simulink model "COMPENSATED"  (R2022b)
settings: Solver=VariableStepAuto  StartTime=0.0  StopTime=0.001  RelTol=1e-3
libraries: spsSeriesRLCBranchLib x9, spsDiodeLib x4, spsIGBTDiodeLib x4, spsCurrentMeasurementLib x3, spsVoltageMeasurementLib x3, spsDCVoltageSourceLib x1, spsPWMGeneratorDCDCLib x1, spspowerguiLib x1
settings Model: Creator=Hafeni  LastModifiedBy=Hafeni

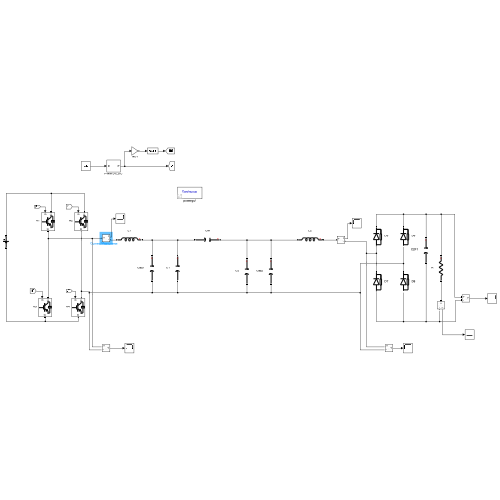
[thumbnail: Simulink's stored preview of the top-level diagram]
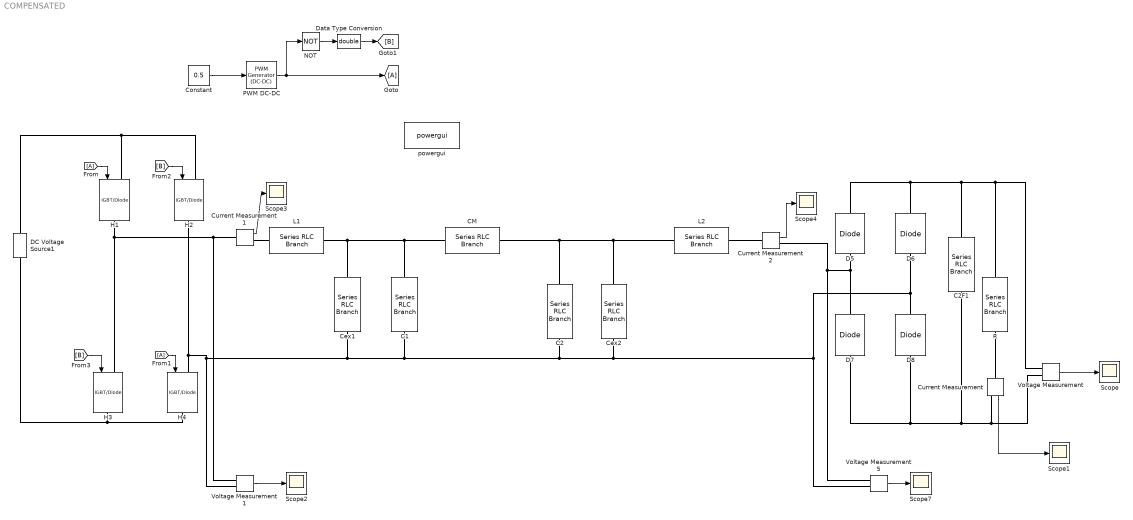
== system COMPENSATED ==
  C1 : spsSeriesRLCBranchLib/Series RLC Branch  LConnTagsString=__new0  RConnTagsString=__new0  BranchType=C  Resistance=1e-6  Inductance=1e-3  SetiL0=off  InitialCurrent=0  Capacitance=1.6460e-12  Setx0=off  InitialVoltage=0  Measurements=Branch voltage
  C2 : spsSeriesRLCBranchLib/Series RLC Branch  LConnTagsString=__new0  RConnTagsString=__new0  BranchType=C  Resistance=1e-6  Inductance=1e-3  SetiL0=off  InitialCurrent=0  Capacitance=1.6456e-12  Setx0=off  InitialVoltage=0  Measurements=Branch voltage
  C2F1 : spsSeriesRLCBranchLib/Series RLC Branch  LConnTagsString=__new0  RConnTagsString=__new0  BranchType=C  Resistance=1e-6  Inductance=1e-3  SetiL0=off  InitialCurrent=0  Capacitance=10e-6  Setx0=off  InitialVoltage=0  Measurements=Branch voltage
  CM : spsSeriesRLCBranchLib/Series RLC Branch  LConnTagsString=__new0  RConnTagsString=__new0  BranchType=C  Resistance=1e-6  Inductance=1e-3  SetiL0=off  InitialCurrent=0  Capacitance=1.0341e-10  Setx0=off  InitialVoltage=0  Measurements=Branch voltage
  Cex1 : spsSeriesRLCBranchLib/Series RLC Branch  LConnTagsString=__new0  RConnTagsString=__new0  BranchType=C  Resistance=1e-6  Inductance=1e-3  SetiL0=off  InitialCurrent=0  Capacitance=100e-12  Setx0=off  InitialVoltage=0  Measurements=Branch voltage
  Cex2 : spsSeriesRLCBranchLib/Series RLC Branch  LConnTagsString=__new0  RConnTagsString=__new0  BranchType=C  Resistance=1e-6  Inductance=1e-3  SetiL0=off  InitialCurrent=0  Capacitance=100e-12  Setx0=off  InitialVoltage=0  Measurements=Branch voltage
  Constant : Constant  Value=0.5
  Current Measurement : spsCurrentMeasurementLib/Current Measurement  PhasorSimulation=off  OutputType=Complex  PSBequivalent=0
  Current Measurement1 : spsCurrentMeasurementLib/Current Measurement  PhasorSimulation=off  OutputType=Complex  PSBequivalent=0
  Current Measurement2 : spsCurrentMeasurementLib/Current Measurement  PhasorSimulation=off  OutputType=Complex  PSBequivalent=0
  D{5..8} (4 alike) : spsDiodeLib/Diode  Ron=0.001  Lon=0  Vf=0.8  IC=0  UseSnubber=0  Rs=500  Cs=250e-9  Measurements=off
  DC Voltage Source1 : spsDCVoltageSourceLib/DC Voltage Source  Amplitude=12  Measurements=None
  Data Type Conversion : DataTypeConversion  OutDataTypeStr=double  SaturateOnIntegerOverflow=off  RndMeth=Floor
  From : From
  From1 : From
  Goto : Goto
  H{1..4} (4 alike) : spsIGBTDiodeLib/IGBT//Diode  Ron=1e-3  Rs=1e5  Cs=inf  Measurements=off
  L1 : spsSeriesRLCBranchLib/Series RLC Branch  LConnTagsString=__new0  RConnTagsString=__new0  BranchType=L  Resistance=1e-6  Inductance=1.38e-6  SetiL0=off  InitialCurrent=0  Capacitance=1.0341e-10  Setx0=off  InitialVoltage=0  Measurements=Branch voltage
  L2 : spsSeriesRLCBranchLib/Series RLC Branch  LConnTagsString=__new0  RConnTagsString=__new0  BranchType=L  Resistance=1e-6  Inductance=1.38e-6  SetiL0=off  InitialCurrent=0  Capacitance=1.0341e-10  Setx0=off  InitialVoltage=0  Measurements=Branch voltage
  "NOT " : Logic  Operator=NOT  IconShape=distinctive  AllPortsSameDT=off  OutDataTypeStr=boolean
  PWM DC-DC : spsPWMGeneratorDCDCLib/PWM Generator (DC-DC)  Fsw=13560000  Ts=0
  R : spsSeriesRLCBranchLib/Series RLC Branch  LConnTagsString=__new0  RConnTagsString=__new0  BranchType=R  Resistance=3.04  Inductance=1e-3  SetiL0=off  InitialCurrent=0  Capacitance=300e-6  Setx0=off  InitialVoltage=0  Measurements=Branch voltage
  Scope{,1..4,7} (6 alike) : Scope
  Voltage Measurement : spsVoltageMeasurementLib/Voltage Measurement  PhasorSimulation=off  OutputType=Complex  PSBequivalent=0
  Voltage Measurement1 : spsVoltageMeasurementLib/Voltage Measurement  PhasorSimulation=off  OutputType=Complex  PSBequivalent=0
  Voltage Measurement5 : spsVoltageMeasurementLib/Voltage Measurement  PhasorSimulation=off  OutputType=Complex  PSBequivalent=0
  powergui : spspowerguiLib/powergui  Priority=1  SimulationMode=Continuous  SampleTime=50e-6  frequency=60  Iterations=50  frequencyindice=0  Pbase=100e6  ErrMax=1e-4  UnitsV=kV  UnitsW=MW  buscounter=0  FunctionMessages=off  echomessages=off  EnableUseOfTLC=off  CurrentSourceSwitches=off  DisableSnubberDevices=off  DisableRonSwitches=off  DisableVfSwitches=off  DisplayEquations=off  AutomaticDiscreteSolvers=off  SolverType=Tustin/Backward Euler (TBE)  Interpol=off  ExternalGateDelay=off  methode=off  Ts=100  x0status=blocks  SPID=on  SwTol=0  HookPort=off  NonlinearTolerance=1e-4  nMaxIteration=100  ContinueOnMaxIteration=off  RestoreLinks=warning  ResistiveCurrentMeasurement=off  Frange=[0:2:500]  Ylog=off  Xlog=on  ShowGrid=off  save=off  variable=ZData  structure=source  ZoomFFT=off  StartTime=0.1  cycles=5  DisplayStyle=2  fundamental=50  FreqAxis=on  MaxFrequency=1000  frequencyindicesteady=1  RmsSteady=1  display=off
  wires:
  Current Measurement/1 -> Scope1/1
  From1/1 -> H4/1
  Voltage Measurement1/1 -> Scope2/1
  From/1 -> H1/1
  "NOT "/1 -> Data Type Conversion/1
  PWM DC-DC/1 -> "NOT "/1, Goto/1
  Constant/1 -> PWM DC-DC/1
  [B] -> H2/1
  [B] -> H3/1
  Current Measurement2/1 -> Scope4/1
  Data Type Conversion/1 -> [B]
  Current Measurement1/1 -> Scope3/1
  Voltage Measurement/1 -> Scope/1
  Voltage Measurement5/1 -> Scope7/1
  connections:
  Voltage Measurement/LConn1 -- C2F1/LConn1 -- D5/RConn1 -- D6/RConn1 -- R/LConn1
  C1/RConn1 -- D6/LConn1 -- D8/RConn1 -- Voltage Measurement5/LConn2 -- Cex2/RConn1 -- C2/RConn1 -- Cex1/RConn1 -- H4/LConn1 -- H2/RConn1 -- Voltage Measurement1/LConn2
  D8/LConn1 -- Voltage Measurement/LConn2 -- Current Measurement/RConn1 -- C2F1/RConn1 -- D7/LConn1
  Current Measurement1/LConn1 -- Voltage Measurement1/LConn1 -- H3/LConn1 -- H1/RConn1
  H4/RConn1 -- DC Voltage Source1/LConn1 -- H3/RConn1
  Current Measurement2/RConn1 -- D7/RConn1 -- D5/LConn1 -- Voltage Measurement5/LConn1
  H1/LConn1 -- H2/LConn1 -- DC Voltage Source1/RConn1
  CM/RConn1 -- C1/LConn1 -- Cex1/LConn1 -- L1/LConn1
  C2/LConn1 -- L2/RConn1 -- Cex2/LConn1 -- CM/LConn1
  Current Measurement/LConn1 -- R/RConn1
  L1/RConn1 -- Current Measurement1/RConn1
  Current Measurement2/LConn1 -- L2/LConn1
